simulink model "ctrl_TAPM"  (R2015a)
settings: Solver=ode3  StartTime=0.0  StopTime=inf  FixedStep=0.01  RelTol=1e-3
values from neighbouring files (symbols this model uses):
  C = [C1;C2;C3;C4;C5;C6]    [initfile.m]    (also in thrustallocationQuadraticFixed.m)
  D = 3.0/100    (= 0.03)    [initfile.m]    (also in thrustallocationQuadraticFixed.m = 0.0411111111111)
  eps_c = 5    [initfile.m]
  epsilon = 0.5    [initfile.m]    (also in thrustallocationPseudo.m = u(10); thrustallocationQuadraticFixed.m = u(10))
  hd = c2d(H1,0.01,'foh')    [initfile.m]
  hd2 = c2d(H2,0.01,'zoh')    [initfile.m]
  I_s = 25000 /747225    (= 0.0334571246947)    [initfile.m]
  k_cc = 1    [initfile.m]
  K_omega = 0.3    [initfile.m]
  K_q1f = 0.0113    [initfile.m]
  K_q1r = K_q1f    (= 0.0113)    [initfile.m]
  K_q2f = 0.0117    [initfile.m]
  K_q2r = K_q2f    (= 0.0117)    [initfile.m]
  K_q3f = 0.0113    [initfile.m]
  K_q3r = K_q3f    (= 0.0113)    [initfile.m]
  K_q4f = 0.0169    [initfile.m]
  K_q4r = K_q4f    (= 0.0169)    [initfile.m]
  K_q5f = 0.0144    [initfile.m]
  K_q5r = K_q5f    (= 0.0144)    [initfile.m]
  K_q6f = 0.0168    [initfile.m]
  K_q6r = K_q6f    (= 0.0168)    [initfile.m]
  K_T1f = 0.3763    [initfile.m]
  K_T1r = K_T1f    (= 0.3763)    [initfile.m]
  K_T2f = 0.3901    [initfile.m]
  K_T2r = K_T2f    (= 0.3901)    [initfile.m]
  K_T3f = 0.3776    [initfile.m]
  K_T3r = K_T3f    (= 0.3776)    [initfile.m]
  K_T4f = 0.5641    [initfile.m]
  K_T4r = K_T4f    (= 0.5641)    [initfile.m]
  K_T5f = 0.4799    [initfile.m]
  K_T5r = K_T5f    (= 0.4799)    [initfile.m]
  K_T6f = 0.5588    [initfile.m]
  K_T6r = K_T6f    (= 0.5588)    [initfile.m]
  Kp = 3.3    [initfile.m]
  Max_Acceleration = 5    [initfile.m]
  Max_rotation = 12*sqrt(lambda)    [initfile.m]
  Max_thrust = 1.5    [initfile.m]
  Min_thrust = -0.8    [initfile.m]
  n_c = 5    [initfile.m]
  p_cc = 0.5    [initfile.m]
  pwm_thr1_backward = coeffvalues(ForceToPWM)    [initfile.m]
  pwm_thr1_forward = coeffvalues(ForceToPWM)    [initfile.m]
  pwm_thr2_backward = coeffvalues(ForceToPWM)    [initfile.m]
  pwm_thr2_forward = coeffvalues(ForceToPWM)    [initfile.m]
  pwm_thr3_backward = coeffvalues(ForceToPWM)    [initfile.m]
  pwm_thr3_forward = coeffvalues(ForceToPWM)    [initfile.m]
  pwm_thr4_backward = coeffvalues(ForceToPWM)    [initfile.m]
  pwm_thr4_forward = coeffvalues(ForceToPWM)    [initfile.m]
  pwm_thr5_backward = coeffvalues(ForceToPWM)    [initfile.m]
  pwm_thr5_forward = coeffvalues(ForceToPWM)    [initfile.m]
  pwm_thr6_backward = coeffvalues(ForceToPWM)    [initfile.m]
  pwm_thr6_forward = coeffvalues(ForceToPWM)    [initfile.m]
  Q_f0 = 0.3    [initfile.m]
  r_cc = 4    [initfile.m]
  Rho = Rho_m    (= 1000)    [initfile.m]
undefined symbols (not defined in the file or in its folder): n_max, Q_max, Thruster
libraries: marine_gnc x10, simulink x6, simulink_extras x3
(part 6 of 6)

== matlab function ctrl_TAPM/TAPM Controller w_observer/LQR/MATLAB Function ==
  data: reset output; timer input; rmax input; y output; eta input
function [reset,y] = fcn(timer,rmax,eta)
persistent controller res tmp

if (isempty(controller))
     controller = 1;
     tmp = 0;
end

res = 0;

pos = sqrt(eta(1)^2+eta(2)^2);

    if pos > rmax && controller ~=2
        controller = 2;
        res = 1;
    elseif pos < 0.9*rmax && timer > 40 && controller ~= 1 && tmp > 190
        controller = 1;
        res = 1;
    end
    
    if pos > rmax 
        res = 1;
        tmp = 0;
    else
        tmp = tmp + 0.01;
    end

    y = controller;
    reset = res;
    
end

== matlab function ctrl_TAPM/TAPM Controller w_observer/LQR/MATLAB Function1 ==
  data: r input; tau output; x_hat input; bias input
function tau = fcn(r,x_hat,bias)

K =[    0.0072          0         0             7.33        0           0
         0              0.0072    -0.0011         0         7.355    0.0195
         0               0          0.72         0           0.0115    10.6236];

P =[    0.0072         0         0
         0    0.0072  -0.0011
         0   0    0.72];

psi = x_hat(3);     

R  = [cos(psi) -sin(psi) 0;
        sin(psi) cos(psi) 0
        0           0      1];     

tau = P*r-K*x_hat;

end
